simulink model "simulink_example"  (Simulink 8.4)
settings: Solver=FixedStepDiscrete  StartTime=0.0  StopTime=inf  FixedStep=Ts  RelTol=1e-3
InitFcn:
  | localName = 'impedance';
  | robotName = 'icubGazeboSim';
  | 
  | Ts = 0.01;
  | ROBOT_DOF = 23;
  | 
  | Kp = 1.5 * ones(ROBOT_DOF, 1);
  | Kd = 0.5 *  ones(ROBOT_DOF, 1);
  | 
  | refMask = zeros(ROBOT_DOF, 1);
  | refMask(4) = 1; %l_shoulder_pitch
  | refMask(7) = 1;
libraries: WBCLibrary x7
settings Model: Creator=makaveli  LastModifiedBy=makaveli
settings DataIOCC: SignalLoggingSaveFormat=Dataset
settings OptimizationCC: ExpressionDepthLimit=128
settings DebuggingCC: UnderspecifiedInitializationDetection=Simplified  MergeDetectMultiDrivingBlocksExec=error  FcnCallInpInsideContextMsg=EnableAllAsError  StateNameClashWarn=none
settings GRTTargetCC: CombineOutputUpdateFcns=on  GRTInterface=off

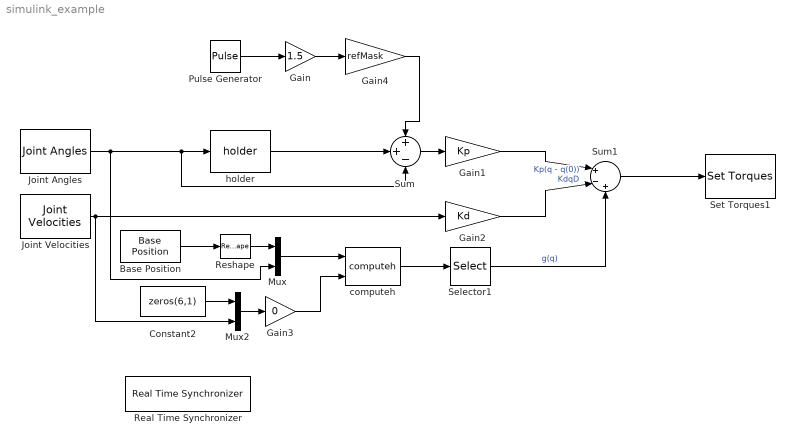
== system simulink_example ==
  Base Position : WBCLibrary/wholeBodyStates/Base Position  robotName=robotName  localName=localName
  Constant2 : Constant  Value=zeros(6,1)
  Gain : Gain  Gain=1.5
  Gain1 : Gain  Gain=Kp
  Gain2 : Gain  Gain=Kd
  Gain3 : Gain  Gain=0
  Gain4 : Gain  Gain=refMask
  Joint Angles : WBCLibrary/wholeBodyStates/Joint Angles  robotName=robotName  localName=localName
  Joint Velocities : WBCLibrary/wholeBodyStates/Joint Velocities  robotName=robotName  localName=localName
  Mux : Mux  Inputs=2
  Mux2 : Mux  Inputs=2
  Pulse Generator : DiscretePulseGenerator  PulseType=Time based  Period=10  PulseWidth=50
  Real Time Synchronizer : WBCLibrary/Utilities/Real Time Synchronizer  Priority=-10  threadPeriod=Ts
  Reshape : Reshape  OutputDimensions=16
  Selector1 : Selector  InputPortWidth=ROBOT_DOF+6  Indices=[7:ROBOT_DOF+6]
  Set Torques1 : WBCLibrary/wholeBodyActuators/Set Torques  val=6  robotName=robotName  localName=localName
  Sum : Sum  Inputs=++-
  Sum1 : Sum  Inputs=|+-+
  computeh : WBCLibrary/wholeBodyModel/Dynamics/computeh  val=7  robotname=robotName  localname=localName
  "holder " : WBCLibrary/Utilities/holder 
  wires:
  Joint Angles/1 -> Sum/3, "holder "/1, Mux/2
  Sum/1 -> Gain1/1
  Gain1/1 -> Sum1/1  "Kp(q - q(0))"
  Gain2/1 -> Sum1/2  "KdqD"
  Gain3/1 -> computeh/2
  computeh/1 -> Selector1/1
  Mux/1 -> computeh/1
  Selector1/1 -> Sum1/3  "g(q)"
  Mux2/1 -> Gain3/1
  Constant2/1 -> Mux2/1
  Joint Velocities/1 -> Gain2/1, Mux2/2
  Sum1/1 -> Set Torques1/1
  Base Position/1 -> Reshape/1
  Reshape/1 -> Mux/1
  Pulse Generator/1 -> Gain/1
  Gain/1 -> Gain4/1
  Gain4/1 -> Sum/1
  "holder "/1 -> Sum/2
